simulink model "helicopter_hat"  (R2021b)
settings: Solver=VariableStepAuto  StartTime=0.0  StopTime=T  RelTol=1e-4
values from neighbouring files (symbols this model uses):
  b = 0.025936940902745    (= 0.0259369409027)    [controller_LQR.m]    (also in controller_check_EKF.m; polish_MPC.m; validation.m)
  K1 = -10.577796958770156    (= -10.5777969588)    [controller_LQR.m]    (also in controller_check_EKF.m; polish_MPC.m; validation.m)
  K3 = -2.433475804656021e-05    (= -2.43347580466e-05)    [controller_LQR.m]    (also in controller_check_EKF.m; polish_MPC.m; validation.m)
  K4 = 5.379206715771331    (= 5.37920671577)    [controller_LQR.m]    (also in controller_check_EKF.m; polish_MPC.m; validation.m)
settings Model: Creator=lcaric  LastModifiedBy=lcaric
settings SolverCC: AlgebraicLoopSolver=TrustRegion
settings DataIOCC: ReturnWorkspaceOutputs=off
settings DebuggingCC: SFMachineParentedDataDiag=warning  ArithmeticOperatorsInVariantConditions=warning
settings SFSimCC: CustomCodeUndefinedFunction=UseInterfaceOnly

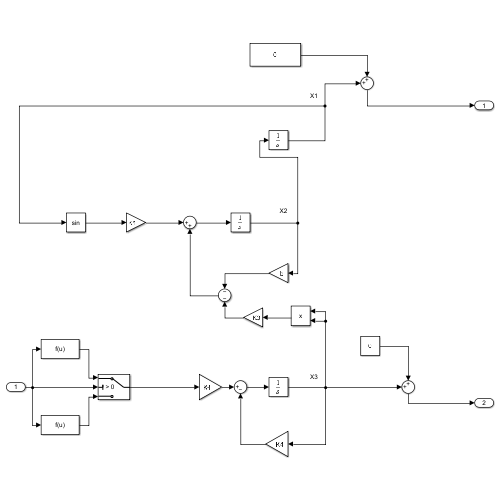
[thumbnail: Simulink's stored preview of the top-level diagram]
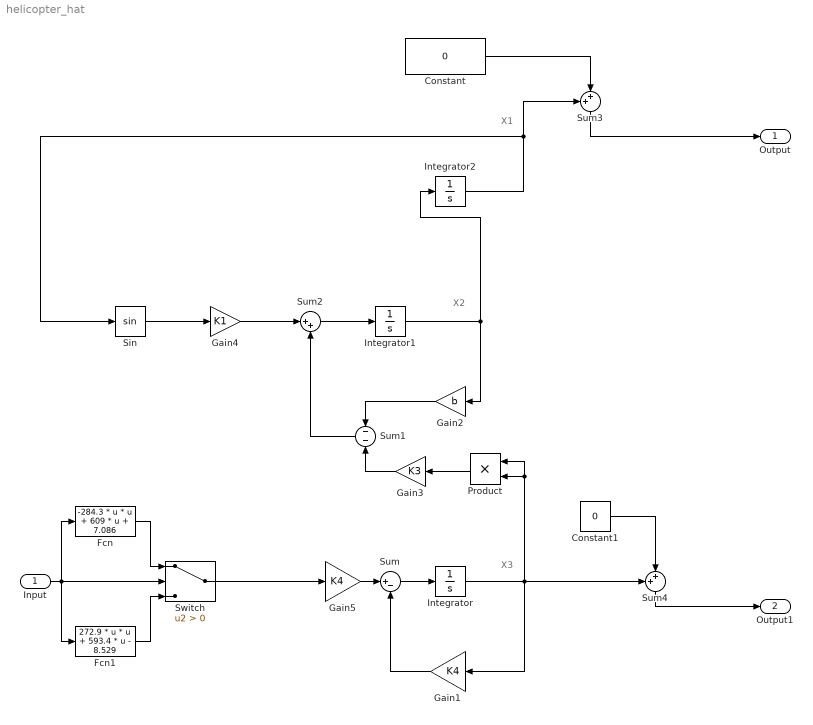
== system helicopter_hat ==
  note: X1
  note: X2
  note: X3
  Input : Inport
  Constant : Constant  Value=0
  Constant1 : Constant  Value=0
  Fcn : Fcn  Expr=-284.3 * u * u + 609 * u + 7.086
  Fcn1 : Fcn  Expr=272.9 * u * u + 593.4 * u - 8.529
  Gain1 : Gain  Gain=K4
  Gain2 : Gain  Gain=b
  Gain3 : Gain  Gain=K3
  Gain4 : Gain  Gain=K1
  Gain5 : Gain  Gain=K4
  Integrator : Integrator
  Integrator1 : Integrator  AbsoluteTolerance=10e-4
  Integrator2 : Integrator
  Product : Product
  Sin : Trigonometry
  Sum : Sum  Inputs=|+-
  Sum1 : Sum  Inputs=--
  Sum2 : Sum  Inputs=|++
  Sum3 : Sum  Inputs=++|
  Sum4 : Sum  Inputs=++|
  Switch : Switch  Criteria=u2 > Threshold
  Output : Outport  VectorParamsAs1DForOutWhenUnconnected=off
  Output1 : Outport  Port=2  VectorParamsAs1DForOutWhenUnconnected=off
  wires:
  Gain1/1 -> Sum/2
  Sum/1 -> Integrator/1
  Integrator/1 -> Gain1/1, Product/2, Product/1, Sum4/1
  Gain2/1 -> Sum1/1
  Gain3/1 -> Sum1/2
  Integrator2/1 -> Sum3/1, Sin/1
  Sum1/1 -> Sum2/2
  Sin/1 -> Gain4/1
  Sum2/1 -> Integrator1/1
  Gain4/1 -> Sum2/1
  Integrator1/1 -> Gain2/1, Integrator2/1
  Sum3/1 -> Output/1
  Constant/1 -> Sum3/2
  Sum4/1 -> Output1/1
  Constant1/1 -> Sum4/2
  Gain5/1 -> Sum/1
  Product/1 -> Gain3/1
  Input/1 -> Fcn1/1, Fcn/1, Switch/2
  Switch/1 -> Gain5/1
  Fcn1/1 -> Switch/3
  Fcn/1 -> Switch/1
